simulink model "tanque_simulink_lineal"  (R2019b)
settings: Solver=VariableStepAuto  StartTime=0.0  StopTime=1500.0  RelTol=1e-3
values from neighbouring files (symbols this model uses):
  A = A /pi^2 /( (rad_menor + h0/tan(ang))^4)    [tanque_simulink_param.m]
  ang = pi/3    (= 1.0471975512)    [tanque_simulink_param.m]
  B = (-sqrt(2*g*h0)*(r_apertura^2)) /( (rad_menor + h0/tan(ang))^2)    [tanque_simulink_param.m]
  C = 1    [tanque_simulink_param.m]
  D = 0    [tanque_simulink_param.m]
  d_p_apertura = 0.05    [tanque_simulink_param.m]
  g = 9.8    [tanque_simulink_param.m]
  h0 = 0.6    [tanque_simulink_param.m]
  p_apertura_lin = Q_ent/(pi*r_apertura^2) / (sqrt(2*g*h0))    [tanque_simulink_param.m]
  Q_ent = 0.0035    [tanque_simulink_param.m]
  r_apertura = 0.0254    [tanque_simulink_param.m]
  rad_menor = 0.05    [tanque_simulink_param.m]
settings Model: Creator=Franco  LastModifiedBy=Franco

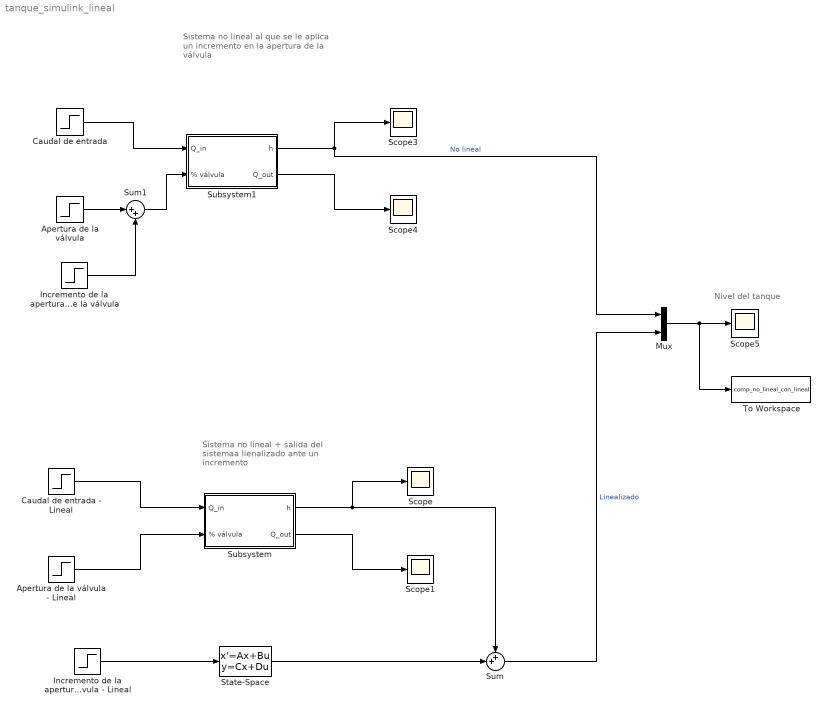
== system tanque_simulink_lineal ==
  note: Nivel del tanque
  note: Sistema no lineal al que se le aplica un incremento en la apertura de la válvula
  note: Sistema no lineal + salida del sistemaa lienalizado ante un incremento
  Apertura de la válvula : Step  After=p_apertura_lin  SampleTime=0
  Apertura de la válvula - Lineal : Step  After=p_apertura_lin  SampleTime=0
  Caudal de entrada : Step  After=Q_ent  SampleTime=0
  Caudal de entrada - Lineal : Step  After=Q_ent  SampleTime=0
  Incremento de la apertura de la válvula : Step  Time=10  After=p_apertura_lin*d_p_apertura  SampleTime=0
  Incremento de la apertura de la válvula - Lineal : Step  Time=10  After=p_apertura_lin *d_p_apertura  SampleTime=0
  Mux : Mux  Inputs=2
  Scope{,1,3..5} (5 alike) : Scope
  State-Space : StateSpace  A=A  B=B  C=C  D=D  InitialCondition=0
  Subsystem : Subsystem
  Subsystem1 : Subsystem
  Sum : Sum  Inputs=++|
  Sum1 : Sum  Inputs=|++
  To Workspace : ToWorkspace  VariableName=comp_no_lineal_con_lineal  SaveFormat=Timeseries  SampleTime=-1
  wires:
  Subsystem/1(h) -> Sum/1, Scope/1
  Subsystem/2(Q_out) -> Scope1/1
  Incremento de la apertura de la válvula - Lineal/1 -> State-Space/1
  State-Space/1 -> Sum/2
  Caudal de entrada/1 -> Subsystem1/1(Q_in)
  Subsystem1/2(Q_out) -> Scope4/1
  Subsystem1/1(h) -> Mux/1, Scope3/1  "No lineal"
  Incremento de la apertura de la válvula/1 -> Sum1/2
  Apertura de la válvula/1 -> Sum1/1
  Sum1/1 -> Subsystem1/2(" % válvula")
  Mux/1 -> To Workspace/1, Scope5/1
  Apertura de la válvula - Lineal/1 -> Subsystem/2(" % válvula")
  Caudal de entrada - Lineal/1 -> Subsystem/1(Q_in)
  Sum/1 -> Mux/2  "Linealizado"

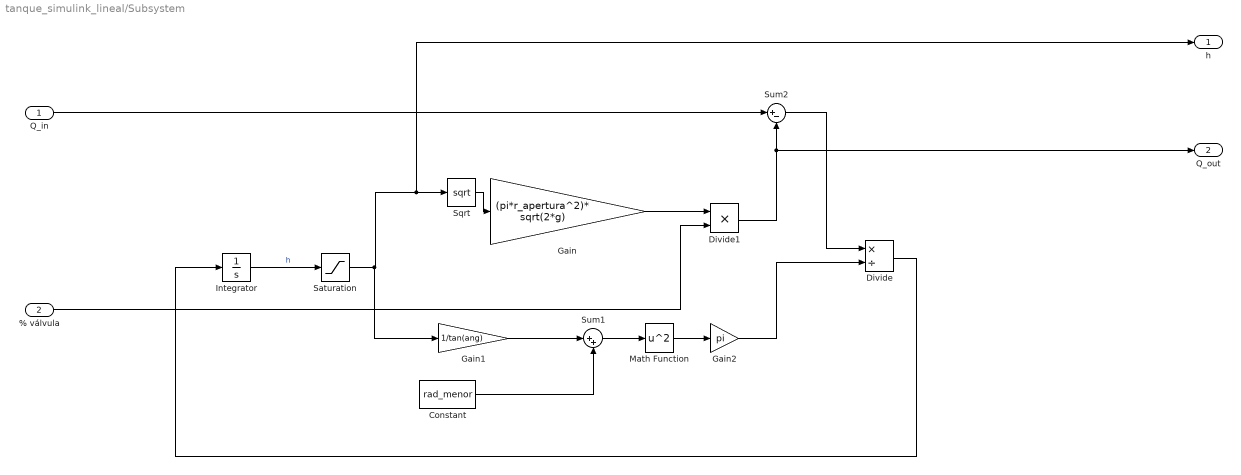
== system tanque_simulink_lineal/Subsystem ==
  Q_in : Inport
  " % válvula" : Inport  Port=2
  Constant : Constant  Value=rad_menor
  Divide : Product  Inputs=*/
  Divide1 : Product  Inputs=**
  Gain : Gain  Gain=(pi*r_apertura^2)* sqrt(2*g)
  Gain1 : Gain  Gain=1/tan(ang)
  Gain2 : Gain  Gain=pi
  Integrator : Integrator  InitialCondition=h0
  Math Function : Math  Operator=square  SignedPower=off  SaturateOnIntegerOverflow=on
  Saturation : Saturate  UpperLimit=1  LowerLimit=0
  Sqrt : Sqrt  SaturateOnIntegerOverflow=on
  Sum1 : Sum  Inputs=|++
  Sum2 : Sum  Inputs=|+-
  h : Outport
  Q_out : Outport  Port=2
  wires:
  Gain/1 -> Divide1/1
  Integrator/1 -> Saturation/1  "h"
  Sqrt/1 -> Gain/1
  Sum2/1 -> Divide/1
  Math Function/1 -> Gain2/1
  Saturation/1 -> Gain1/1, h/1, Sqrt/1
  Gain1/1 -> Sum1/1
  Sum1/1 -> Math Function/1
  Divide/1 -> Integrator/1
  Gain2/1 -> Divide/2
  Q_in/1 -> Sum2/1
  Constant/1 -> Sum1/2
  " % válvula"/1 -> Divide1/2
  Divide1/1 -> Q_out/1, Sum2/2

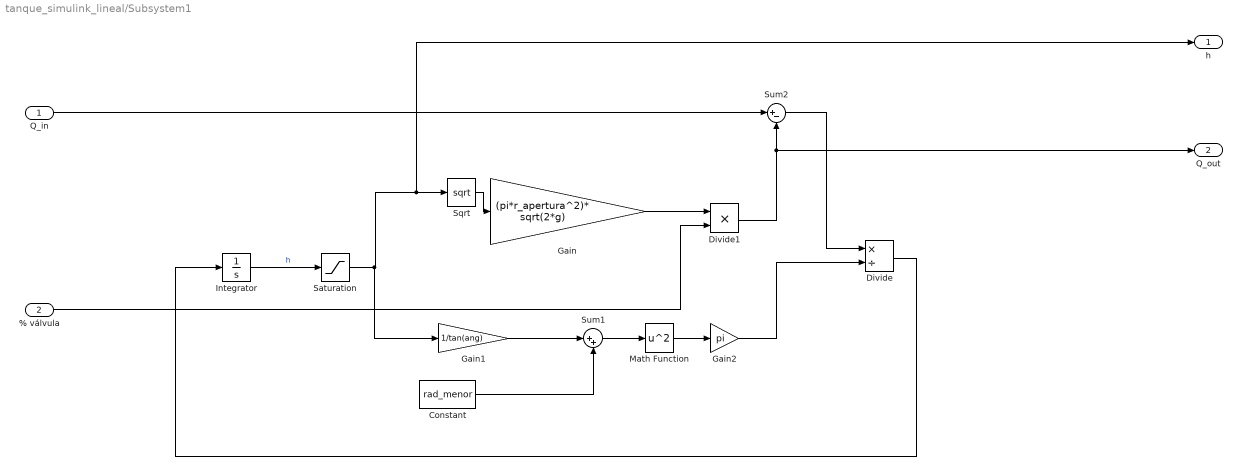
== system tanque_simulink_lineal/Subsystem1 ==
  Q_in : Inport
  " % válvula" : Inport  Port=2
  Constant : Constant  Value=rad_menor
  Divide : Product  Inputs=*/
  Divide1 : Product  Inputs=**
  Gain : Gain  Gain=(pi*r_apertura^2)* sqrt(2*g)
  Gain1 : Gain  Gain=1/tan(ang)
  Gain2 : Gain  Gain=pi
  Integrator : Integrator  InitialCondition=h0
  Math Function : Math  Operator=square  SignedPower=off  SaturateOnIntegerOverflow=on
  Saturation : Saturate  UpperLimit=1  LowerLimit=0
  Sqrt : Sqrt  SaturateOnIntegerOverflow=on
  Sum1 : Sum  Inputs=|++
  Sum2 : Sum  Inputs=|+-
  h : Outport
  Q_out : Outport  Port=2
  wires:
  Gain/1 -> Divide1/1
  Integrator/1 -> Saturation/1  "h"
  Sqrt/1 -> Gain/1
  Sum2/1 -> Divide/1
  Math Function/1 -> Gain2/1
  Saturation/1 -> Gain1/1, h/1, Sqrt/1
  Gain1/1 -> Sum1/1
  Sum1/1 -> Math Function/1
  Divide/1 -> Integrator/1
  Gain2/1 -> Divide/2
  Q_in/1 -> Sum2/1
  Constant/1 -> Sum1/2
  " % válvula"/1 -> Divide1/2
  Divide1/1 -> Q_out/1, Sum2/2
